simulink model "chirp_excite_controlled"  (R2012b)
settings: Solver=FixedStepDiscrete  StartTime=0.0  StopTime=Tfinal  RelTol=1e-3
values from neighbouring files (symbols this model uses):
  Kd = c2d(Krob,Ts)    [run_autonomous_control.m]
  Ts = 0.001    [run_autonomous_control.m]
undefined symbols (not defined in the file or in its folder): AMP1, AMP2, KON, National_Instruments, PCI, T, Tfinal
libraries: rtwinlib x2, simulink x1
settings Model: SimulationMode=external  ExtModeTrigDuration=1000000  ExtModeArchiveMode=auto  ExtModeArchiveFileName=dataarch  ExtModeArchiveDirName=.\  Creator=f.cardoso-ribeiro  LastModifiedBy=f.cardoso-ribeiro
settings SolverCC: AutoInsertRateTranBlk=on
settings DataIOCC: LimitDataPoints=off  SaveOutput=off  SignalLogging=off  DSMLogging=off  SaveTime=off
settings HardwareCC: ProdIntDivRoundTo=Zero  ProdEndianess=LittleEndian  ProdHWDeviceType=Generic->32-bit x86 compatible
settings RTWCC: SystemTargetFile=rtwin.tlc  TemplateMakefile=rtwin.tmf  Description=Real-Time Windows Target  RTWVerbose=off  ProcessScript=rtwin_make_rtw_hook  RTWCompilerOptimization=On
settings CodeAppCC: MaxIdLength=95
settings RTWinTargetCC: TargetLibSuffix=_rtwin.lib  TargetPreCompLibLocation=C:\Program Files\MATLAB\R2012b\toolbox\rtw\targets\rtwin\lib\win64  CodeReplacementLibrary=ANSI_C  RTWinDir=C:/PROGRA~1/MATLAB/R2012b/toolbox/rtw/targets/rtwin  TargetArch=win64

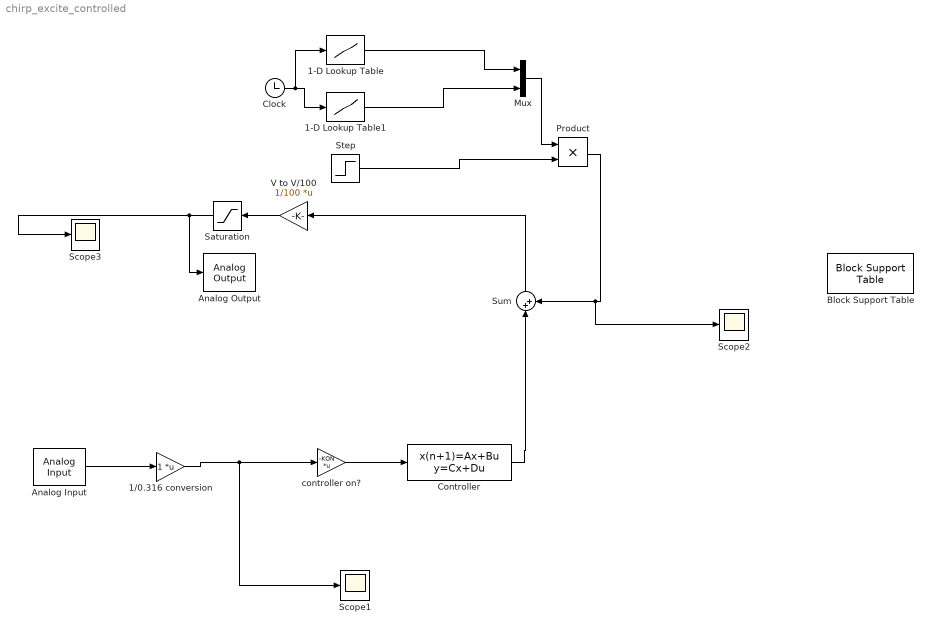
== system chirp_excite_controlled ==
  1-D Lookup Table : Lookup_n-D  NumberOfTableDimensions=1  BreakpointsForDimension1=T  Table=AMP1  RndMeth=Simplest  InputSameDT=on
  1-D Lookup Table1 : Lookup_n-D  NumberOfTableDimensions=1  BreakpointsForDimension1=T  Table=AMP2  RndMeth=Simplest  InputSameDT=on
  1/0.316 conversion : Gain  Multiplication=Matrix(K*u)
  Analog Input : rtwinlib/Analog Input  SampleTime=Ts  MaxMissedTicks=10  ShowMissedTicks=off  YieldWhenWaiting=off  DrvName=National_Instruments/PCI-6024E  DrvAddress=4294967295  DrvOptions=[1 0 0 0 0 0]  Channels=[1 2]  RangeMode=1  VoltRange=2  DataType=1
      settings: AttributesFormatString=National Instruments\nPCI-6024E [auto]
  Analog Output : rtwinlib/Analog Output  SampleTime=Ts  MaxMissedTicks=10  ShowMissedTicks=off  YieldWhenWaiting=off  DrvName=National_Instruments/PCI-6024E  DrvAddress=4294967295  DrvOptions=[1 0 0 0 0 0]  Channels=[1 2]  RangeMode=1  VoltRange=1  InitialValue=0  FinalValue=0
      settings: AttributesFormatString=National Instruments\nPCI-6024E [auto]
  Block Support Table : simulink/Model-Wide Utilities/Block Support Table
  Clock : Clock
  Controller : DiscreteStateSpace  A=Kd.A  B=Kd.B  C=Kd.C  D=Kd.D  SampleTime=Ts
  Mux : Mux  Inputs=2
  Product : Product  RndMeth=Zero
  Saturation : Saturate  UpperLimit=1.5  LowerLimit=-1.5
  Scope1 : Scope
      settings: TimeRange=240  YMin=-0.6  YMax=0.7  SaveName=output
  Scope2 : Scope
      settings: YMin=-70  YMax=70  SaveName=input
  Scope3 : Scope
      settings: TimeRange=240  YMin=-1.5  YMax=1.5  SaveName=control_input
  Step : Step  Time=Tfinal-20  Before=1  After=0  SampleTime=0
  Sum : Sum  Inputs=|++
  "V to V/100 " : Gain  Gain=1/100  Multiplication=Matrix(K*u)
  controller on? : Gain  Gain=-KON  Multiplication=Matrix(K*u)
  wires:
  Analog Input/1 -> 1/0.316 conversion/1
  "V to V/100 "/1 -> Saturation/1
  controller on?/1 -> Controller/1
  Controller/1 -> Sum/1
  Step/1 -> Product/2
  1-D Lookup Table/1 -> Mux/1
  1-D Lookup Table1/1 -> Mux/2
  Mux/1 -> Product/1
  Clock/1 -> 1-D Lookup Table/1, 1-D Lookup Table1/1
  Sum/1 -> "V to V/100 "/1
  Product/1 -> Scope2/1, Sum/2
  Saturation/1 -> Analog Output/1, Scope3/1
  1/0.316 conversion/1 -> Scope1/1, controller on?/1
